simulink model "wlan_phy_tx_pmd"  (Simulink 7.8)
settings: Solver=VariableStepDiscrete  SolverMode=SingleTasking  StartTime=0.0  StopTime=inf  RelTol=1e-3
PostLoadFcn:
  | wlan_phy_tx_init
InitFcn:
  | wlan_phy_tx_init
StartFcn:
  | wlan_phy_tx_init
undefined symbols (not defined in the file): gcbh, ht_preamble_rom, MAX_CP_LEN, MAX_DATA_BITS_PER_SYM_PERIOD, MAX_NCBPS, MAX_NUM_BYTES, MAX_NUM_SC, MAX_NUM_SYMS, mcs_rom_11ag, mcs_rom_11n, Mod_Constellation_16QAM, Mod_Constellation_64QAM, Mod_Constellation_BPSK, Mod_Constellation_QPSK, Preamble_IQ, Preamble_IQ_scaled, tx_sim, wlan_tx_interleave_rom, xlBlockLoadCallback, xlGetNormalizedPeriod
libraries: xbsIndex_r4 x1358, xbsEDKLib_r4 x1
(part 8 of 10)

== system wlan_phy_tx_pmd/PSDU Syms Gen/Modulate/Control & Pilots/Data SC Map ==
  note: ROMs store mapping of subcarrier indexes as used by
      | upstream logic to subcarrier indexes into the IFFT. These
      | maps also encode which subcarriers are occupied.
      | Unoccupied subcarrier indexes are encoded as 64 in the
      | ROM (64 is an invalid subcarrier index).
      |
      | The mapping in these ROMs implements the effective
      | 'fftshift' from the 802.11 standard, where subcarriers are
      | loaded starting from the most negative subcarrier.
  Full Rate : Inport
  sc_ind : Inport  Port=2
  11a Subcarrier Map : xbsIndex_r4/ROM  depth=MAX_NUM_SC  initVector=sc_data_sym_map_11a  distributed_mem=Distributed memory  rst=off  init_reg=0  en=off  latency=0  gui_display_data_type=Fixed-point  arith_type=Unsigned  n_bits=ceil(log2(MAX_NUM_SC))+1  bin_pt=0  preci_type=Single  exp_width=8  frac_width=24  dbl_ovrd=off  optimize=Area  use_rpm=on  block_type=sprom
  11n HT20 Subcarrier Map : xbsIndex_r4/ROM  depth=MAX_NUM_SC  initVector=sc_data_sym_map_11n  distributed_mem=Distributed memory  rst=off  init_reg=0  en=off  latency=0  gui_display_data_type=Fixed-point  arith_type=Unsigned  n_bits=ceil(log2(MAX_NUM_SC))+1  bin_pt=0  preci_type=Single  exp_width=8  frac_width=24  dbl_ovrd=off  optimize=Area  use_rpm=on  block_type=sprom
  Constant2 : xbsIndex_r4/Constant  const=MAX_NUM_SC  gui_display_data_type=Fixed-point  arith_type=Unsigned  n_bits=ceil(log2(MAX_NUM_SC))+1  bin_pt=0  preci_type=Single  exp_width=8  frac_width=24  explicit_period=off  period=1  equ=P=C  opselect=C  inp2=PCIN>>17  opr=+  inp1=P  carry=CIN  dbl_ovrd=off  block_type=constant
  Logical : xbsIndex_r4/Logical  logical_function=AND  inputs=2  en=off  latency=0  precision=Full  arith_type=Unsigned  n_bits=16  bin_pt=0  align_bp=on  dbl_ovrd=off  block_type=logical
  Mux1 : xbsIndex_r4/Mux  inputs=2  en=off  latency=0  precision=Full  arith_type=Unsigned  n_bits=16  bin_pt=14  quantization=Truncate  overflow=Wrap  dbl_ovrd=off  block_type=mux
  Relational1 : xbsIndex_r4/Relational  mode=a!=b  en=off  latency=0  dbl_ovrd=off  block_type=relational
  Slice : xbsIndex_r4/Slice  nbits=ceil(log2(MAX_NUM_SC))  boolean_output=off  mode=Lower Bit Location + Width  bit1=0  base1=MSB of Input  bit0=0  base0=LSB of Input  dbl_ovrd=off  block_type=slice
  data_sym_ind : Outport
  data_sym_valid : Outport  Port=2
  wires:
  sc_ind/1 -> 11a Subcarrier Map/1, 11n HT20 Subcarrier Map/1
  Constant2/1 -> Relational1/2
  11a Subcarrier Map/1 -> Mux1/2
  11n HT20 Subcarrier Map/1 -> Mux1/3
  Logical/1 -> Mux1/1
  Mux1/1 -> Relational1/1, Slice/1
  Relational1/1 -> data_sym_valid/1
  [Tx_PHY_Mode_11n] -> Logical/1
  Full Rate/1 -> Logical/2
  Slice/1 -> data_sym_ind/1

== system wlan_phy_tx_pmd/PSDU Syms Gen/Modulate/Control & Pilots/Pilot Gen ==
  sc_ind : Inport
  reset : Inport  Port=2
  Pilot Shift : Inport  Port=3
  Constant1 : xbsIndex_r4/Constant  const=Mod_Constellation_BPSK(1)  gui_display_data_type=Fixed-point  arith_type=Signed (2's comp)  n_bits=12  bin_pt=11  preci_type=Single  exp_width=8  frac_width=24  explicit_period=off  period=1  equ=P=C  opselect=C  inp2=PCIN>>17  opr=+  inp1=P  carry=CIN  dbl_ovrd=off  block_type=constant
  Constant5 : xbsIndex_r4/Constant  const=Mod_Constellation_BPSK(2)  gui_display_data_type=Fixed-point  arith_type=Signed (2's comp)  n_bits=12  bin_pt=11  preci_type=Single  exp_width=8  frac_width=24  explicit_period=off  period=1  equ=P=C  opselect=C  inp2=PCIN>>17  opr=+  inp1=P  carry=CIN  dbl_ovrd=off  block_type=constant
  Delay : xbsIndex_r4/Delay  rst=off  infoeditControl=Selection of Reset will increase slice count due to use of real FFs and instead of SRLs  en=off  latency=1  dbl_ovrd=off  reg_retiming=off  block_type=delay
  Logical : xbsIndex_r4/Logical  logical_function=XOR  inputs=2  en=off  latency=0  precision=Full  arith_type=Unsigned  n_bits=8  bin_pt=2  align_bp=on  dbl_ovrd=off  block_type=logical
      settings: xl_area=[0, 0, 0, 0, 0, 0, 0]  block_version=VER_STRING_GOES_HERE
  Mux1 : xbsIndex_r4/Mux  inputs=2  en=off  latency=0  precision=Full  arith_type="Signed  (2's comp)"  n_bits=8  bin_pt=2  quantization=Truncate  overflow=Wrap  dbl_ovrd=off  block_type=mux
      settings: xl_area=[16 0 0 32 0 0 0]  block_version=VER_STRING_GOES_HERE
  Pilot Selection : Subsystem
  Posedge : Subsystem
  Relational1 : xbsIndex_r4/Relational  mode=a<b  en=off  latency=0  dbl_ovrd=off  block_type=relational
  Scrambling LFSR : Subsystem
  pilot_valid : Outport
  Pilot_I : Outport  Port=2
  wires:
  Pilot Selection/1(Pilot) -> pilot_valid/1
  Pilot Selection/2(Negate) -> Logical/1
  sc_ind/1 -> Pilot Selection/1(sc_ind), Delay/1, Relational1/1
  Delay/1 -> Relational1/2
  Relational1/1 -> Posedge/1(D)
  Posedge/1(Q) -> Scrambling LFSR/1(en)
  Scrambling LFSR/1(Q) -> Logical/2
  Logical/1 -> Mux1/1
  Constant5/1 -> Mux1/2
  Constant1/1 -> Mux1/3
  Mux1/1 -> Pilot_I/1
  reset/1 -> Scrambling LFSR/2(rst)
  Pilot Shift/1 -> Pilot Selection/2(Shift)

== system wlan_phy_tx_pmd/PSDU Syms Gen/Modulate/Control & Pilots/Posedge ==
  note: Rising Edge Detection
  D : Inport
  Delay : xbsIndex_r4/Delay  rst=off  infoeditControl=Selection of Reset will increase slice count due to use of real FFs and instead of SRLs  en=off  latency=1  dbl_ovrd=off  reg_retiming=off  block_type=delay
      settings: infoedit=Hardware notes: A delay line is a chain, each link of which is an SRL16 followed by a flip-flop. If register retiming is enabled, the delay line is a chain of flip-flops.  xl_area=[1 1 0 0 0 0 0]  block_version=VER_STRING_GOES_HERE
  Inverter : xbsIndex_r4/Inverter  en=off  latency=0  dbl_ovrd=off  block_type=inv
      settings: xl_area=[0 0 0 0 0 0 0]  block_version=VER_STRING_GOES_HERE
  Logical1 : xbsIndex_r4/Logical  logical_function=AND  inputs=2  en=off  latency=0  precision=Full  arith_type=Unsigned  n_bits=8  bin_pt=2  align_bp=on  dbl_ovrd=off  block_type=logical
      settings: xl_area=[1 0 0 1 0 0 0]  block_version=VER_STRING_GOES_HERE
  Q : Outport
  wires:
  D/1 -> Logical1/2, Delay/1
  Logical1/1 -> Q/1
  Inverter/1 -> Logical1/1
  Delay/1 -> Inverter/1

== system wlan_phy_tx_pmd/PSDU Syms Gen/Modulate/Control & Pilots/Posedge1 ==
  note: Rising Edge Detection
  D : Inport
  Delay : xbsIndex_r4/Delay  rst=off  infoeditControl=Selection of Reset will increase slice count due to use of real FFs and instead of SRLs  en=off  latency=1  dbl_ovrd=off  reg_retiming=off  block_type=delay
      settings: infoedit=Hardware notes: A delay line is a chain, each link of which is an SRL16 followed by a flip-flop. If register retiming is enabled, the delay line is a chain of flip-flops.  xl_area=[1 1 0 0 0 0 0]  block_version=VER_STRING_GOES_HERE
  Inverter : xbsIndex_r4/Inverter  en=off  latency=0  dbl_ovrd=off  block_type=inv
      settings: xl_area=[0 0 0 0 0 0 0]  block_version=VER_STRING_GOES_HERE
  Logical1 : xbsIndex_r4/Logical  logical_function=AND  inputs=2  en=off  latency=0  precision=Full  arith_type=Unsigned  n_bits=8  bin_pt=2  align_bp=on  dbl_ovrd=off  block_type=logical
      settings: xl_area=[1 0 0 1 0 0 0]  block_version=VER_STRING_GOES_HERE
  Q : Outport
  wires:
  Delay/1 -> Inverter/1
  Inverter/1 -> Logical1/1
  Logical1/1 -> Q/1
  D/1 -> Delay/1, Logical1/2

== system wlan_phy_tx_pmd/PSDU Syms Gen/Modulate/Control & Pilots/S-R Latch1 ==
  S : Inport
  R : Inport  Port=2
  Constant1 : xbsIndex_r4/Constant  const=1  gui_display_data_type=Fixed-point  arith_type=Boolean  n_bits=1  bin_pt=0  preci_type=Single  exp_width=8  frac_width=24  explicit_period=off  period=1  equ=P=C  opselect=C  inp2=PCIN>>17  opr=+  inp1=P  carry=CIN  dbl_ovrd=off  block_type=constant
      settings: block_version=VER_STRING_GOES_HERE
  Convert1 : xbsIndex_r4/Convert  gui_display_data_type=Boolean  arith_type=Boolean  n_bits=1  bin_pt=0  float_type=Single  exp_bits=8  fraction_bits=24  quantization=Truncate  overflow=Wrap  en=off  latency=0  dbl_ovrd=off  pipeline=off  block_type=convert
  Convert2 : xbsIndex_r4/Convert  gui_display_data_type=Boolean  arith_type=Boolean  n_bits=1  bin_pt=0  float_type=Single  exp_bits=8  fraction_bits=24  quantization=Truncate  overflow=Wrap  en=off  latency=0  dbl_ovrd=off  pipeline=off  block_type=convert
  Register2 : xbsIndex_r4/Register  init=0  rst=on  en=on  dbl_ovrd=off  block_type=register
      settings: xl_area=[1 1 0 0 0 0 0]  block_version=VER_STRING_GOES_HERE
  Q : Outport
  wires:
  Convert2/1 -> Register2/3
  Convert1/1 -> Register2/2
  Constant1/1 -> Register2/1
  R/1 -> Convert1/1
  Register2/1 -> Q/1
  S/1 -> Convert2/1

== system wlan_phy_tx_pmd/PSDU Syms Gen/Modulate/Control & Pilots/Subcarrier Index Count ==
  en : Inport
  reset : Inport  Port=2
  AddSub : xbsIndex_r4/AddSub  mode=Subtraction  use_carryin=off  use_carryout=off  en=off  latency=0  precision=Full  arith_type=Unsigned  n_bits=16  bin_pt=14  quantization=Truncate  overflow=Wrap  dbl_ovrd=off  use_behavioral_HDL=off  hw_selection=Fabric  pipelined=off  block_type=addsub
  Constant1 : xbsIndex_r4/Constant  const=1  gui_display_data_type=Fixed-point  arith_type=Unsigned  n_bits=1  bin_pt=0  preci_type=Single  exp_width=8  frac_width=24  explicit_period=off  period=1  equ=P=C  opselect=C  inp2=PCIN>>17  opr=+  inp1=P  carry=CIN  dbl_ovrd=off  block_type=constant
  Logical1 : xbsIndex_r4/Logical  logical_function=AND  inputs=2  en=off  latency=0  precision=Full  arith_type=Unsigned  n_bits=16  bin_pt=0  align_bp=on  dbl_ovrd=off  block_type=logical
  Logical2 : xbsIndex_r4/Logical  logical_function=OR  inputs=2  en=off  latency=0  precision=Full  arith_type=Unsigned  n_bits=16  bin_pt=0  align_bp=on  dbl_ovrd=off  block_type=logical
  Relational3 : xbsIndex_r4/Relational  mode=a=b  en=off  latency=0  dbl_ovrd=off  block_type=relational
  Subcarrier Index : xbsIndex_r4/Counter  cnt_type=Free Running  cnt_to=47  operation=Up  start_count=0  cnt_by_val=1  arith_type=Unsigned  n_bits=ceil(log2(MAX_NUM_SC))  bin_pt=0  load_pin=off  rst=on  en=on  explicit_period=off  period=4  dbl_ovrd=off  use_behavioral_HDL=off  implementation=Fabric  block_type=counter
  sc_ind : Outport
  last : Outport  Port=2
  wires:
  Subcarrier Index/1 -> Relational3/2, sc_ind/1
  AddSub/1 -> Relational3/1
  Relational3/1 -> Logical1/1
  en/1 -> Subcarrier Index/2, Logical1/2
  Logical2/1 -> Subcarrier Index/1
  reset/1 -> Logical2/1
  Logical1/1 -> Logical2/2, last/1
  [regTx_NUM_SC] -> AddSub/1
  Constant1/1 -> AddSub/2

== system wlan_phy_tx_pmd/PSDU Syms Gen/Pkt Data/BRAM IF 64b/BRAM Addr Map ==
  note: OFDM Byte Index Tx -> Memory mapping
      | 11a/g Tx
      |
      | T=Tx byte index
      | M=Memory byte index
      |
      | T  M
      | 0  0   SIGNAL[0]
      | 1  1   SIGNAL[1]
      | 2  2   SIGNAL[2]
      | 3  3   SERVICE[0]
      | 4  4   SERVICE[1]
      |    5   no read
      |    ...
      |    15   no read
      | 5  16  MPDU[0]
      | 6  17  MPDU[1]
      | ...
  note: OFDM Byte Index Tx -> Memory mapping
      | 11n/ac Tx
      |
      | T=Rx byte index
      | M=Memory byte index
      |
      | T  M
      | 0  0   SIGNAL[0]
      | 1  1   SIGNAL[1]
      | 2  2   SIGNAL[2]
      | 3  3   HT-SIG[0]
      | 4  4   HT-SIG[1]
      | 5  5   HT-SIG[2]
      | 6  6   HT-SIG[3]
      | 7  7   HT-SIG[4]
      | 8  8   HT-SIG[5]
      | 9  9   SERVICE[0]
      | 10 10  SERVICE[1]
      |    11  no read
      | ...
      |    15  no read
      | 11 16  MAC Payload[0]
      | 12 17  MAC Payload[1]
      | ...
  note: Packet buffer contents depend on the PHY mode. 11n payloads
      | must include the HTSIG field, for example. For easier addressing
      | in software the Tx PHY logic uses the address mapping below. Note
      | that the MAC payload always starts at a 64-bit aligned address. This
      | allows efficient use of the DMA in CPU high to move MAC payloads into
      | the packet buffer. CPU Low adds the PHY-mode-specific fields before
      | transmission.
      |
      | The MAC code must write valid bytes for SIGNAL, HT-SIG and SERVICE
      | fields. The PHY will abort if the SIGNAL or HT-SIG fields are invlid.
      | The MAC software must set the SERVICE field bytes to 0 to ensure
      | the resulting payload can be de-scrambled by the receiver.
  Tx Ind : Inport
  AddSub1 : xbsIndex_r4/AddSub  mode=Addition  use_carryin=off  use_carryout=off  en=off  latency=0  precision=User Defined  arith_type=Unsigned  n_bits=ceil(log2(MAX_NUM_BYTES))  bin_pt=0  quantization=Truncate  overflow=Wrap  dbl_ovrd=off  use_behavioral_HDL=off  hw_selection=Fabric  pipelined=off  block_type=addsub
  Constant1 : xbsIndex_r4/Constant  const=4  gui_display_data_type=Fixed-point  arith_type=Unsigned  n_bits=3  bin_pt=0  preci_type=Single  exp_width=8  frac_width=24  explicit_period=off  period=1  equ=P=C  opselect=C  inp2=PCIN>>17  opr=+  inp1=P  carry=CIN  dbl_ovrd=off  block_type=constant
  Constant2 : xbsIndex_r4/Constant  const=11  gui_display_data_type=Fixed-point  arith_type=Unsigned  n_bits=4  bin_pt=0  preci_type=Single  exp_width=8  frac_width=24  explicit_period=off  period=1  equ=P=C  opselect=C  inp2=PCIN>>17  opr=+  inp1=P  carry=CIN  dbl_ovrd=off  block_type=constant
  Constant3 : xbsIndex_r4/Constant  const=10  gui_display_data_type=Fixed-point  arith_type=Unsigned  n_bits=4  bin_pt=0  preci_type=Single  exp_width=8  frac_width=24  explicit_period=off  period=1  equ=P=C  opselect=C  inp2=PCIN>>17  opr=+  inp1=P  carry=CIN  dbl_ovrd=off  block_type=constant
  Constant4 : xbsIndex_r4/Constant  const=5  gui_display_data_type=Fixed-point  arith_type=Unsigned  n_bits=3  bin_pt=0  preci_type=Single  exp_width=8  frac_width=24  explicit_period=off  period=1  equ=P=C  opselect=C  inp2=PCIN>>17  opr=+  inp1=P  carry=CIN  dbl_ovrd=off  block_type=constant
  Mux1 : xbsIndex_r4/Mux  inputs=2  en=off  latency=0  precision=Full  arith_type=Unsigned  n_bits=16  bin_pt=14  quantization=Truncate  overflow=Wrap  dbl_ovrd=off  block_type=mux
  Mux2 : xbsIndex_r4/Mux  inputs=2  en=off  latency=0  precision=Full  arith_type=Unsigned  n_bits=16  bin_pt=14  quantization=Truncate  overflow=Wrap  dbl_ovrd=off  block_type=mux
  Mux5 : xbsIndex_r4/Mux  inputs=2  en=off  latency=0  precision=Full  arith_type=Unsigned  n_bits=16  bin_pt=14  quantization=Truncate  overflow=Wrap  dbl_ovrd=off  block_type=mux
  Relational : xbsIndex_r4/Relational  mode=a<=b  en=off  latency=0  dbl_ovrd=off  block_type=relational
  Mem Addr : Outport
  wires:
  Mux2/1 -> AddSub1/2
  Tx Ind/1 -> Relational/1, AddSub1/1, Mux5/3
  Relational/1 -> Mux5/1
  Mux5/1 -> Mem Addr/1
  AddSub1/1 -> Mux5/2
  [Tx_PHY_Mode_11n_ac] -> Mux1/1, Mux2/1
  Constant1/1 -> Mux1/2
  Mux1/1 -> Relational/2
  Constant2/1 -> Mux2/2
  Constant3/1 -> Mux1/3
  Constant4/1 -> Mux2/3

== system wlan_phy_tx_pmd/PSDU Syms Gen/Pkt Data/BRAM IF 64b/BRAM Interface ==
  Pkt Buf Index : Inport
  64b Word Addr : Inport  Port=2
  BRAM_Addr : xbsIndex_r4/Gateway Out  inherit_from_input=off  hdl_port=on  timing_constraint=None  locs_specified=off  LOCs={}  UseAsDAC=off  DACChannel='1'  block_type=gatewayout
      settings: infoedit="Gateway out block.  Converts Xilinx fixed point inputs into ouputs of type Simulink integer, double, or fixed point.<P><P>Hardware notes:  In hardware these blocks become top level output ports or are discarded, depending on how they are configured."  xl_area=[0, 0, 0, 0, 0, 0, 0]  block_version=VER_STRING_GOES_HERE
  BRAM_Din : xbsIndex_r4/Gateway In  gui_display_data_type=Fixed-point  arith_type=Unsigned  n_bits=64  bin_pt=0  preci_type=Single  exp_width=8  frac_width=24  quantization="Round  (unbiased: +/- Inf)"  overflow=Saturate  period=1  dbl_ovrd=off  timing_constraint=None  locs_specified=off  LOCs={}  UseAsADC=off  ADCChannel='1'  inherit_from_input=off  hdl_port=on  block_type=gatewayin
      settings: block_version=VER_STRING_GOES_HERE
  BRAM_Dout : xbsIndex_r4/Gateway Out  inherit_from_input=off  hdl_port=on  timing_constraint=None  locs_specified=off  LOCs={}  UseAsDAC=off  DACChannel='1'  block_type=gatewayout
      settings: infoedit="Gateway out block.  Converts Xilinx fixed point inputs into ouputs of type Simulink integer, double, or fixed point.<P><P>Hardware notes:  In hardware these blocks become top level output ports or are discarded, depending on how they are configured."  xl_area=[0, 0, 0, 0, 0, 0, 0]  block_version=VER_STRING_GOES_HERE
  BRAM_En : xbsIndex_r4/Gateway Out  inherit_from_input=off  hdl_port=on  timing_constraint=None  locs_specified=off  LOCs={}  UseAsDAC=off  DACChannel='1'  block_type=gatewayout
      settings: infoedit="Gateway out block.  Converts Xilinx fixed point inputs into ouputs of type Simulink integer, double, or fixed point.<P><P>Hardware notes:  In hardware these blocks become top level output ports or are discarded, depending on how they are configured."  block_version=8.2.02
  BRAM_Reset : xbsIndex_r4/Gateway Out  inherit_from_input=off  hdl_port=on  timing_constraint=None  locs_specified=off  LOCs={}  UseAsDAC=off  DACChannel='1'  block_type=gatewayout
      settings: infoedit="Gateway out block.  Converts Xilinx fixed point inputs into ouputs of type Simulink integer, double, or fixed point.<P><P>Hardware notes:  In hardware these blocks become top level output ports or are discarded, depending on how they are configured."  block_version=8.2.02
  BRAM_WEn : xbsIndex_r4/Gateway Out  inherit_from_input=off  hdl_port=on  timing_constraint=None  locs_specified=off  LOCs={}  UseAsDAC=off  DACChannel='1'  block_type=gatewayout
      settings: infoedit="Gateway out block.  Converts Xilinx fixed point inputs into ouputs of type Simulink integer, double, or fixed point.<P><P>Hardware notes:  In hardware these blocks become top level output ports or are discarded, depending on how they are configured."  xl_area=[0, 0, 0, 0, 0, 0, 0]  block_version=VER_STRING_GOES_HERE
  Concat : xbsIndex_r4/Concat  num_inputs=4  dbl_ovrd=off  block_type=concat
  Constant : Constant  Value=0
  Constant1 : xbsIndex_r4/Constant  const=1  gui_display_data_type=Fixed-point  arith_type=Unsigned  n_bits=1  bin_pt=0  preci_type=Single  exp_width=8  frac_width=24  explicit_period=on  period=1  equ=P=C  opselect=C  inp2=PCIN>>17  opr=+  inp1=P  carry=CIN  dbl_ovrd=off  block_type=constant
      settings: block_version=8.2.02
  Constant2 : xbsIndex_r4/Constant  const=0  gui_display_data_type=Fixed-point  arith_type=Unsigned  n_bits=1  bin_pt=0  preci_type=Single  exp_width=8  frac_width=24  explicit_period=on  period=1  equ=P=C  opselect=C  inp2=PCIN>>17  opr=+  inp1=P  carry=CIN  dbl_ovrd=off  block_type=constant
      settings: block_version=8.2.02
  Constant3 : xbsIndex_r4/Constant  const=0  gui_display_data_type=Fixed-point  arith_type=Unsigned  n_bits=3  bin_pt=0  preci_type=Single  exp_width=8  frac_width=24  explicit_period=off  period=1  equ=P=C  opselect=C  inp2=PCIN>>17  opr=+  inp1=P  carry=CIN  dbl_ovrd=off  block_type=constant
  Constant4 : xbsIndex_r4/Constant  const=0  gui_display_data_type=Fixed-point  arith_type=Unsigned  n_bits=16  bin_pt=0  preci_type=Single  exp_width=8  frac_width=24  explicit_period=off  period=1  equ=P=C  opselect=C  inp2=PCIN>>17  opr=+  inp1=P  carry=CIN  dbl_ovrd=off  block_type=constant
  Constant7 : xbsIndex_r4/Constant  const=0  gui_display_data_type=Fixed-point  arith_type=Unsigned  n_bits=64  bin_pt=0  preci_type=Single  exp_width=8  frac_width=24  explicit_period=on  period=1  equ=P=C  opselect=C  inp2=PCIN>>17  opr=+  inp1=P  carry=CIN  dbl_ovrd=off  block_type=constant
      settings: block_version=8.2.02
  Constant8 : xbsIndex_r4/Constant  const=0  gui_display_data_type=Fixed-point  arith_type=Unsigned  n_bits=8  bin_pt=0  preci_type=Single  exp_width=8  frac_width=24  explicit_period=on  period=1  equ=P=C  opselect=C  inp2=PCIN>>17  opr=+  inp1=P  carry=CIN  dbl_ovrd=off  block_type=constant
      settings: block_version=8.2.02
  Sim RAM : Subsystem
  Simulation Multiplexer : xbsIndex_r4/Simulation Multiplexer  sim_sel=1  hw_sel=2  block_type=simmux
      settings: infoedit="Distinguish input subsystems as \"simulation only\" and \"generation only\".  The input specified For Simulation will be used during Simulink simulation.  The input specified For Generation will be used during code generation.  This block will typically be used on the output of a HW Co-Simulation, Black Box, or ModelSim subsystem.<br><br>Hardware Notes: This block costs nothing."
  Terminator{,2..5} (5 alike) : Terminator
  64b Data : Outport
  wires:
  Sim RAM/1(64b) -> Simulation Multiplexer/1
  BRAM_Din/1 -> Simulation Multiplexer/2
  BRAM_WEn/1 -> Terminator5/1
  BRAM_Reset/1 -> Terminator4/1
  BRAM_En/1 -> Terminator3/1
  BRAM_Dout/1 -> Terminator2/1
  BRAM_Addr/1 -> Terminator/1
  Constant2/1 -> BRAM_Reset/1
  Constant1/1 -> BRAM_En/1
  Constant/1 -> BRAM_Din/1
  Constant7/1 -> BRAM_Dout/1
  Constant8/1 -> BRAM_WEn/1
  64b Word Addr/1 -> Sim RAM/1(Addr), Concat/3
  Constant3/1 -> Concat/4
  Constant4/1 -> Concat/1
  Concat/1 -> BRAM_Addr/1
  Simulation Multiplexer/1 -> 64b Data/1
  Pkt Buf Index/1 -> Concat/2

== system wlan_phy_tx_pmd/PSDU Syms Gen/Pkt Data/BRAM IF 64b/Byte Sel ==
  64b : Inport
  B Sel : Inport  Port=2
  B0 : xbsIndex_r4/Slice  nbits=8  boolean_output=off  mode=Lower Bit Location + Width  bit1=0  base1=MSB of Input  bit0=0  base0=LSB of Input  dbl_ovrd=off  block_type=slice
  B1 : xbsIndex_r4/Slice  nbits=8  boolean_output=off  mode=Lower Bit Location + Width  bit1=0  base1=MSB of Input  bit0=8  base0=LSB of Input  dbl_ovrd=off  block_type=slice
  B2 : xbsIndex_r4/Slice  nbits=8  boolean_output=off  mode=Lower Bit Location + Width  bit1=0  base1=MSB of Input  bit0=16  base0=LSB of Input  dbl_ovrd=off  block_type=slice
  B3 : xbsIndex_r4/Slice  nbits=8  boolean_output=off  mode=Lower Bit Location + Width  bit1=0  base1=MSB of Input  bit0=24  base0=LSB of Input  dbl_ovrd=off  block_type=slice
  B4 : xbsIndex_r4/Slice  nbits=8  boolean_output=off  mode=Lower Bit Location + Width  bit1=0  base1=MSB of Input  bit0=32  base0=LSB of Input  dbl_ovrd=off  block_type=slice
  B5 : xbsIndex_r4/Slice  nbits=8  boolean_output=off  mode=Lower Bit Location + Width  bit1=0  base1=MSB of Input  bit0=40  base0=LSB of Input  dbl_ovrd=off  block_type=slice
  B6 : xbsIndex_r4/Slice  nbits=8  boolean_output=off  mode=Lower Bit Location + Width  bit1=0  base1=MSB of Input  bit0=48  base0=LSB of Input  dbl_ovrd=off  block_type=slice
  B7 : xbsIndex_r4/Slice  nbits=8  boolean_output=off  mode=Lower Bit Location + Width  bit1=0  base1=MSB of Input  bit0=56  base0=LSB of Input  dbl_ovrd=off  block_type=slice
  Mux : xbsIndex_r4/Mux  inputs=8  en=off  latency=0  precision=Full  arith_type=Unsigned  n_bits=16  bin_pt=14  quantization=Truncate  overflow=Wrap  dbl_ovrd=off  block_type=mux
  B : Outport
  wires:
  Mux/1 -> B/1
  B Sel/1 -> Mux/1
  64b/1 -> B2/1, B3/1, B4/1, B5/1, B6/1, B7/1, B1/1, B0/1
  B3/1 -> Mux/5
  B2/1 -> Mux/4
  B1/1 -> Mux/3
  B0/1 -> Mux/2
  B4/1 -> Mux/6
  B5/1 -> Mux/7
  B6/1 -> Mux/8
  B7/1 -> Mux/9

== system wlan_phy_tx_pmd/PSDU Syms Gen/Pkt Data/FCS Calc/Byte Sel ==
  32b : Inport
  B Sel : Inport  Port=2
  B0 : xbsIndex_r4/Slice  nbits=8  boolean_output=off  mode=Lower Bit Location + Width  bit1=0  base1=MSB of Input  bit0=0  base0=LSB of Input  dbl_ovrd=off  block_type=slice
  B1 : xbsIndex_r4/Slice  nbits=8  boolean_output=off  mode=Lower Bit Location + Width  bit1=0  base1=MSB of Input  bit0=8  base0=LSB of Input  dbl_ovrd=off  block_type=slice
  B2 : xbsIndex_r4/Slice  nbits=8  boolean_output=off  mode=Lower Bit Location + Width  bit1=0  base1=MSB of Input  bit0=16  base0=LSB of Input  dbl_ovrd=off  block_type=slice
  B3 : xbsIndex_r4/Slice  nbits=8  boolean_output=off  mode=Lower Bit Location + Width  bit1=0  base1=MSB of Input  bit0=24  base0=LSB of Input  dbl_ovrd=off  block_type=slice
  Constant : xbsIndex_r4/Constant  const=hex2dec('87654321') %hex2dec('FF00FF00') %  gui_display_data_type=Fixed-point  arith_type=Unsigned  n_bits=32  bin_pt=0  preci_type=Single  exp_width=8  frac_width=24  explicit_period=on  period=1  equ=P=C  opselect=C  inp2=PCIN>>17  opr=+  inp1=P  carry=CIN  dbl_ovrd=off  block_type=constant
  Mux : xbsIndex_r4/Mux  inputs=4  en=off  latency=0  precision=Full  arith_type=Unsigned  n_bits=16  bin_pt=14  quantization=Truncate  overflow=Wrap  dbl_ovrd=off  block_type=mux
  B : Outport
  wires:
  Mux/1 -> B/1
  B Sel/1 -> Mux/1
  32b/1 -> B0/1, B1/1, B2/1, B3/1
  B0/1 -> Mux/5
  B1/1 -> Mux/4
  B2/1 -> Mux/3
  B3/1 -> Mux/2

== system wlan_phy_tx_pmd/PSDU Syms Gen/Pkt Data/FCS Calc/CRC32 Calc ==
  byte : Inport
  en : Inport  Port=2
  24LSB : xbsIndex_r4/Slice  nbits=24  boolean_output=off  mode=Lower Bit Location + Width  bit1=0  base1=MSB of Input  bit0=0  base0=LSB of Input  dbl_ovrd=off  block_type=slice
      settings: infoedit="Extracts a given range of bits from each input sample and presents it at the output.  The output type is ordinarily unsigned with binary point at zero, but can be Boolean when the slice is one bit wide.<P><P>Hardware notes: In hardware this block costs nothing."  block_version=VER_STRING_GOES_HERE
  8MSB : xbsIndex_r4/Slice  nbits=8  boolean_output=off  mode=Upper Bit Location + Width  bit1=0  base1=MSB of Input  bit0=0  base0=LSB of Input  dbl_ovrd=off  block_type=slice
      settings: infoedit="Extracts a given range of bits from each input sample and presents it at the output.  The output type is ordinarily unsigned with binary point at zero, but can be Boolean when the slice is one bit wide.<P><P>Hardware notes: In hardware this block costs nothing."  block_version=VER_STRING_GOES_HERE
  Assert : xbsIndex_r4/Assert  assert_type=off  type_source=Explicitly  gui_display_data_type=Fixed-point  arith_type="Signed  (2's comp)"  n_bits=16  bin_pt=14  preci_type=Single  exp_width=8  frac_width=24  assert_rate=on  rate_source=Explicitly  period=1  output_port=on  block_type=assert
  Assert1 : xbsIndex_r4/Assert  assert_type=off  type_source=Explicitly  gui_display_data_type=Fixed-point  arith_type="Signed  (2's comp)"  n_bits=16  bin_pt=14  preci_type=Single  exp_width=8  frac_width=24  assert_rate=on  rate_source=Explicitly  period=1  output_port=on  block_type=assert
      settings: block_version=VER_STRING_GOES_HERE
  B0 : xbsIndex_r4/Slice  nbits=8  boolean_output=off  mode=Lower Bit Location + Width  bit1=0  base1=MSB of Input  bit0=0  base0=LSB of Input  dbl_ovrd=off  block_type=slice
  B1 : xbsIndex_r4/Slice  nbits=8  boolean_output=off  mode=Lower Bit Location + Width  bit1=0  base1=MSB of Input  bit0=8  base0=LSB of Input  dbl_ovrd=off  block_type=slice
  B2 : xbsIndex_r4/Slice  nbits=8  boolean_output=off  mode=Lower Bit Location + Width  bit1=0  base1=MSB of Input  bit0=16  base0=LSB of Input  dbl_ovrd=off  block_type=slice
  B3 : xbsIndex_r4/Slice  nbits=8  boolean_output=off  mode=Lower Bit Location + Width  bit1=0  base1=MSB of Input  bit0=24  base0=LSB of Input  dbl_ovrd=off  block_type=slice
  CRC Remainders1 : xbsIndex_r4/ROM  depth=256  initVector=CRC_Table32  distributed_mem=Distributed memory  rst=off  init_reg=0  en=off  latency=0  gui_display_data_type=Fixed-point  arith_type=Unsigned  n_bits=32  bin_pt=0  preci_type=Single  exp_width=8  frac_width=24  dbl_ovrd=off  optimize=Area  use_rpm=off  block_type=sprom
      settings: xl_area=[0, 0, 0, 0, 0, 0, 0]  block_version=VER_STRING_GOES_HERE
  Concat : xbsIndex_r4/Concat  num_inputs=4  dbl_ovrd=off  block_type=concat
  Concat1 : xbsIndex_r4/Concat  num_inputs=2  dbl_ovrd=off  block_type=concat
      settings: block_version=VER_STRING_GOES_HERE
  Constant1 : xbsIndex_r4/Constant  const=0  gui_display_data_type=Fixed-point  arith_type=Unsigned  n_bits=8  bin_pt=0  preci_type=Single  exp_width=8  frac_width=24  explicit_period=off  period=1  equ=P=C  opselect=C  inp2=PCIN>>17  opr=+  inp1=P  carry=CIN  dbl_ovrd=off  block_type=constant
      settings: block_version=VER_STRING_GOES_HERE
  Endian Swap : Subsystem
  Endian Swap1 : Subsystem
  Endian Swap2 : Subsystem
  Endian Swap3 : Subsystem
  Endian Swap4 : Subsystem
  Inverter : xbsIndex_r4/Inverter  en=off  latency=0  dbl_ovrd=off  block_type=inv
  Logical3 : xbsIndex_r4/Logical  logical_function=XOR  inputs=2  en=off  latency=0  precision=Full  arith_type=Unsigned  n_bits=8  bin_pt=2  align_bp=on  dbl_ovrd=off  block_type=logical
      settings: xl_area=[0, 0, 0, 0, 0, 0, 0]  block_version=VER_STRING_GOES_HERE
  Logical4 : xbsIndex_r4/Logical  logical_function=XOR  inputs=2  en=off  latency=0  precision=Full  arith_type=Unsigned  n_bits=8  bin_pt=2  align_bp=on  dbl_ovrd=off  block_type=logical
      settings: xl_area=[0, 0, 0, 0, 0, 0, 0]  block_version=VER_STRING_GOES_HERE
  crc_accum : xbsIndex_r4/Register  init=hex2dec('FFFFFFFF')  rst=on  en=on  dbl_ovrd=off  block_type=register
      settings: xl_area=[0, 0, 0, 0, 0, 0, 0]  block_version=VER_STRING_GOES_HERE
  CRC32 : Outport
  wires:
  Inverter/1 -> B0/1, B1/1, B3/1, B2/1
  Endian Swap4/1(I) -> Concat/4
  Endian Swap3/1(I) -> Concat/3
  Endian Swap2/1(I) -> Concat/2
  Endian Swap1/1(I) -> Concat/1
  Endian Swap/1(I) -> Logical3/2
  Concat/1 -> Assert/1
  B3/1 -> Endian Swap4/1(B)
  B2/1 -> Endian Swap3/1(B)
  B1/1 -> Endian Swap2/1(B)
  B0/1 -> Endian Swap1/1(B)
  byte/1 -> Endian Swap/1(B)
  8MSB/1 -> Logical3/1
  24LSB/1 -> Concat1/1
  [TX_RESET] -> crc_accum/2
  Assert1/1 -> Inverter/1, 8MSB/1, 24LSB/1
  crc_accum/1 -> Assert1/1
  Logical4/1 -> crc_accum/1
  Constant1/1 -> Concat1/2
  Concat1/1 -> Logical4/1
  CRC Remainders1/1 -> Logical4/2
  Logical3/1 -> CRC Remainders1/1
  Assert/1 -> CRC32/1
  en/1 -> crc_accum/3

== system wlan_phy_tx_pmd/PSDU Syms Gen/Pkt Data/FCS Calc/posedge ==
  D : Inport
  Delay : xbsIndex_r4/Delay  rst=off  infoeditControl=Selection of Reset will increase slice count due to use of real FFs and instead of SRLs  en=off  latency=1  dbl_ovrd=off  reg_retiming=off  block_type=delay
      settings: infoedit=Hardware notes: A delay line is a chain, each link of which is an SRL16 followed by a flip-flop. If register retiming is enabled, the delay line is a chain of flip-flops.  xl_area=[1 1 0 0 0 0 0]  block_version=VER_STRING_GOES_HERE
  Inverter : xbsIndex_r4/Inverter  en=off  latency=0  dbl_ovrd=off  block_type=inv
      settings: xl_area=[0 0 0 0 0 0 0]  block_version=VER_STRING_GOES_HERE
  Logical1 : xbsIndex_r4/Logical  logical_function=AND  inputs=2  en=off  latency=0  precision=Full  arith_type=Unsigned  n_bits=8  bin_pt=2  align_bp=on  dbl_ovrd=off  block_type=logical
      settings: xl_area=[1 0 0 1 0 0 0]  block_version=VER_STRING_GOES_HERE
  Q : Outport
  wires:
  Logical1/1 -> Q/1
  D/1 -> Delay/1, Logical1/1
  Delay/1 -> Inverter/1
  Inverter/1 -> Logical1/2

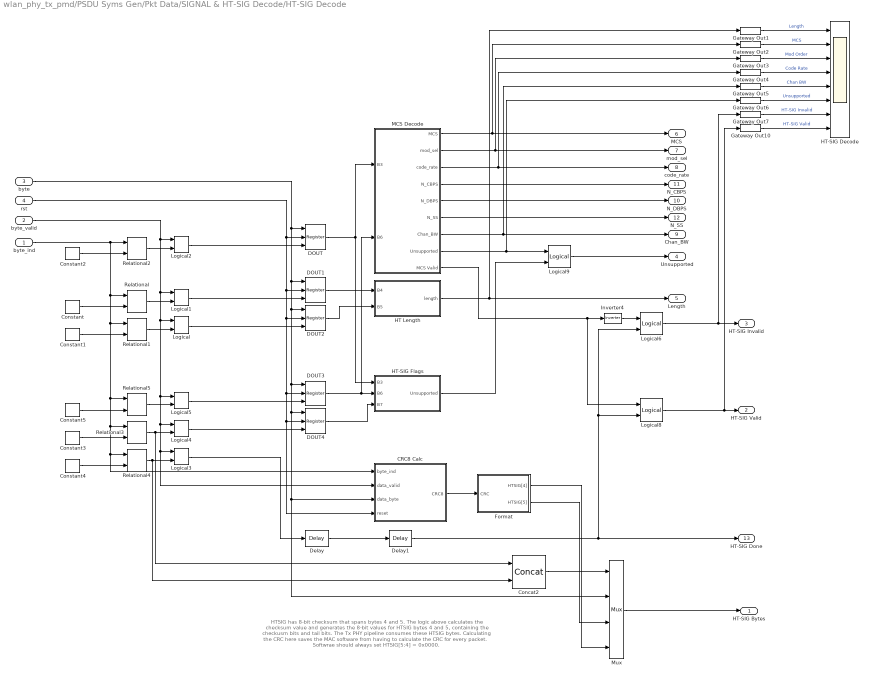
== system wlan_phy_tx_pmd/PSDU Syms Gen/Pkt Data/SIGNAL & HT-SIG Decode/HT-SIG Decode ==
  note: HTSIG has 8-bit checksum that spans bytes 4 and 5. The logic above
      | calculates the checksum value and generates the 8-bit values for HTSIG
      | bytes 4 and 5, containing the checkusm bits and tail bits. The Tx PHY
      | pipeline consumes these HTSIG bytes. Calculating the CRC here saves
      | the MAC software from having to calculate the CRC for every packet.
      |
      | Softwrae should always set HTSIG[5:4] = 0x0000.
  byte_ind : Inport
  byte_valid : Inport  Port=2
  byte : Inport  Port=3
  rst : Inport  Port=4
  CRC8 Calc : Subsystem
  Concat2 : xbsIndex_r4/Concat  num_inputs=2  dbl_ovrd=off  block_type=concat
  Constant : xbsIndex_r4/Constant  const=4  gui_display_data_type=Fixed-point  arith_type=Unsigned  n_bits=3  bin_pt=0  preci_type=Single  exp_width=8  frac_width=24  explicit_period=off  period=1  equ=P=C  opselect=C  inp2=PCIN>>17  opr=+  inp1=P  carry=CIN  dbl_ovrd=off  block_type=constant
  Constant1 : xbsIndex_r4/Constant  const=5  gui_display_data_type=Fixed-point  arith_type=Unsigned  n_bits=3  bin_pt=0  preci_type=Single  exp_width=8  frac_width=24  explicit_period=off  period=1  equ=P=C  opselect=C  inp2=PCIN>>17  opr=+  inp1=P  carry=CIN  dbl_ovrd=off  block_type=constant
  Constant2 : xbsIndex_r4/Constant  const=3  gui_display_data_type=Fixed-point  arith_type=Unsigned  n_bits=2  bin_pt=0  preci_type=Single  exp_width=8  frac_width=24  explicit_period=off  period=1  equ=P=C  opselect=C  inp2=PCIN>>17  opr=+  inp1=P  carry=CIN  dbl_ovrd=off  block_type=constant
  Constant3 : xbsIndex_r4/Constant  const=7  gui_display_data_type=Fixed-point  arith_type=Unsigned  n_bits=3  bin_pt=0  preci_type=Single  exp_width=8  frac_width=24  explicit_period=off  period=1  equ=P=C  opselect=C  inp2=PCIN>>17  opr=+  inp1=P  carry=CIN  dbl_ovrd=off  block_type=constant
  Constant4 : xbsIndex_r4/Constant  const=8  gui_display_data_type=Fixed-point  arith_type=Unsigned  n_bits=4  bin_pt=0  preci_type=Single  exp_width=8  frac_width=24  explicit_period=off  period=1  equ=P=C  opselect=C  inp2=PCIN>>17  opr=+  inp1=P  carry=CIN  dbl_ovrd=off  block_type=constant
  Constant5 : xbsIndex_r4/Constant  const=6  gui_display_data_type=Fixed-point  arith_type=Unsigned  n_bits=3  bin_pt=0  preci_type=Single  exp_width=8  frac_width=24  explicit_period=off  period=1  equ=P=C  opselect=C  inp2=PCIN>>17  opr=+  inp1=P  carry=CIN  dbl_ovrd=off  block_type=constant
  DOUT : xbsIndex_r4/Register  init=0  rst=on  en=on  dbl_ovrd=off  block_type=register
  DOUT1 : xbsIndex_r4/Register  init=100  rst=on  en=on  dbl_ovrd=off  block_type=register
  DOUT2 : xbsIndex_r4/Register  init=0  rst=on  en=on  dbl_ovrd=off  block_type=register
  DOUT3 : xbsIndex_r4/Register  init=hex2dec('03')  rst=on  en=on  dbl_ovrd=off  block_type=register
  DOUT4 : xbsIndex_r4/Register  init=hex2dec('E0')  rst=on  en=on  dbl_ovrd=off  block_type=register
  Delay : xbsIndex_r4/Delay  rst=off  infoeditControl=Selection of Reset will increase slice count due to use of real FFs and instead of SRLs  en=off  latency=1  dbl_ovrd=off  reg_retiming=off  block_type=delay
  Delay1 : xbsIndex_r4/Delay  rst=off  infoeditControl=Selection of Reset will increase slice count due to use of real FFs and instead of SRLs  en=off  latency=1  dbl_ovrd=off  reg_retiming=off  block_type=delay
  Format : Subsystem
  Gateway Out{1..7,10} (8 alike) : xbsIndex_r4/Gateway Out  inherit_from_input=off  hdl_port=off  timing_constraint=None  locs_specified=off  LOCs={}  UseAsDAC=off  DACChannel='1'  block_type=gatewayout
  HT Length : Subsystem
  HT-SIG Decode : Scope  NumInputPorts=8
      settings: TimeRange=7000  YMin=0~0~0~0~100~-1~-1~-1  YMax=1~1~150~1~300~1~1~1  SaveName=ScopeData45
  HT-SIG Flags : Subsystem
  Inverter4 : xbsIndex_r4/Inverter  en=off  latency=0  dbl_ovrd=off  block_type=inv
  Logical{,1..6,8} (8 alike) : xbsIndex_r4/Logical  logical_function=AND  inputs=2  en=off  latency=0  precision=Full  arith_type=Unsigned  n_bits=16  bin_pt=0  align_bp=on  dbl_ovrd=off  block_type=logical
  Logical9 : xbsIndex_r4/Logical  logical_function=OR  inputs=2  en=off  latency=0  precision=Full  arith_type=Unsigned  n_bits=16  bin_pt=0  align_bp=on  dbl_ovrd=off  block_type=logical
  MCS Decode : Subsystem
  Mux : xbsIndex_r4/Mux  inputs=3  en=off  latency=0  precision=Full  arith_type=Unsigned  n_bits=16  bin_pt=14  quantization=Truncate  overflow=Wrap  dbl_ovrd=off  block_type=mux
  Relational{,1..5} (6 alike) : xbsIndex_r4/Relational  mode=a=b  en=off  latency=0  dbl_ovrd=off  block_type=relational
  HT-SIG Bytes : Outport
  HT-SIG Valid : Outport  Port=2
  HT-SIG Invalid : Outport  Port=3
  Unsupported : Outport  Port=4
  Length : Outport  Port=5
  MCS : Outport  Port=6
  mod_sel : Outport  Port=7
  code_rate : Outport  Port=8
  Chan_BW : Outport  Port=9
  N_DBPS : Outport  Port=10
  N_CBPS : Outport  Port=11
  N_SS : Outport  Port=12
  HT-SIG Done : Outport  Port=13
  wires:
  rst/1 -> DOUT1/2, DOUT2/2, DOUT3/2, DOUT4/2, CRC8 Calc/4(reset), DOUT/2
  Logical1/1 -> DOUT1/3
  Logical2/1 -> DOUT/3
  Logical/1 -> DOUT2/3
  Relational/1 -> Logical1/2
  Relational2/1 -> Logical2/2
  Relational1/1 -> Logical/2
  Constant2/1 -> Relational2/2
  Constant1/1 -> Relational1/2
  Constant/1 -> Relational/2
  byte/1 -> DOUT1/1, DOUT2/1, DOUT4/1, CRC8 Calc/3(data_byte), Mux/2, DOUT3/1, DOUT/1
  byte_ind/1 -> Relational/1, Relational1/1, Relational3/1, Relational4/1, CRC8 Calc/1(byte_ind), Relational5/1, Relational2/1
  byte_valid/1 -> Logical1/1, Logical/1, Logical4/1, Logical3/1, CRC8 Calc/2(data_valid), Logical5/1, Logical2/1
  Logical4/1 -> DOUT4/3
  Logical5/1 -> DOUT3/3
  Logical3/1 -> Delay/1
  Relational3/1 -> Logical4/2, Concat2/1
  Relational5/1 -> Logical5/2
  Relational4/1 -> Logical3/2, Concat2/2
  Constant5/1 -> Relational5/2
  Constant4/1 -> Relational4/2
  Constant3/1 -> Relational3/2
  DOUT/1 -> HT-SIG Flags/1(B3), MCS Decode/1(B3)
  DOUT1/1 -> HT Length/1(B4)
  DOUT2/1 -> HT Length/2(B5)
  DOUT3/1 -> HT-SIG Flags/2(B6), MCS Decode/2(B6)
  Gateway Out1/1 -> HT-SIG Decode/1  "Length"
  Gateway Out10/1 -> HT-SIG Decode/8  "HT-SIG Valid"
  Gateway Out2/1 -> HT-SIG Decode/2  "MCS"
  Gateway Out3/1 -> HT-SIG Decode/3  "Mod Order"
  Gateway Out4/1 -> HT-SIG Decode/4  "Code Rate"
  MCS Decode/1(MCS) -> MCS/1, Gateway Out2/1
  MCS Decode/2(mod_sel) -> mod_sel/1, Gateway Out3/1
  MCS Decode/3(code_rate) -> code_rate/1, Gateway Out4/1
  MCS Decode/4(N_CBPS) -> N_CBPS/1
  MCS Decode/5(N_DBPS) -> N_DBPS/1
  MCS Decode/6(N_SS) -> N_SS/1
  MCS Decode/7(Chan_BW) -> Chan_BW/1, Gateway Out5/1
  HT Length/1(length) -> Length/1, Gateway Out1/1
  Logical6/1 -> HT-SIG Invalid/1, Gateway Out7/1
  Logical8/1 -> HT-SIG Valid/1, Gateway Out10/1
  Delay/1 -> Delay1/1
  HT-SIG Flags/1(Unsupported) -> Logical9/2
  MCS Decode/8(Unsupported) -> Gateway Out6/1, Logical9/1
  Gateway Out5/1 -> HT-SIG Decode/5  "Chan BW"
  Gateway Out6/1 -> HT-SIG Decode/6  "Unsupported"
  Delay1/1 -> HT-SIG Done/1, Logical8/2, Logical6/2
  DOUT4/1 -> HT-SIG Flags/3(B7)
  Logical9/1 -> Unsupported/1
  Gateway Out7/1 -> HT-SIG Decode/7  "HT-SIG Invalid"
  Inverter4/1 -> Logical6/1
  Mux/1 -> HT-SIG Bytes/1
  Concat2/1 -> Mux/1
  MCS Decode/9(MCS Valid) -> Inverter4/1, Logical8/1
  CRC8 Calc/1(CRC8) -> Format/1(CRC)
  Format/2(HTSIG[5]) -> Mux/3
  Format/1(HTSIG[4]) -> Mux/4

== system wlan_phy_tx_pmd/PSDU Syms Gen/Pkt Data/SIGNAL & HT-SIG Decode/S-R Latch1 ==
  S : Inport
  R : Inport  Port=2
  Constant1 : xbsIndex_r4/Constant  const=1  gui_display_data_type=Fixed-point  arith_type=Boolean  n_bits=1  bin_pt=0  preci_type=Single  exp_width=8  frac_width=24  explicit_period=off  period=1  equ=P=C  opselect=C  inp2=PCIN>>17  opr=+  inp1=P  carry=CIN  dbl_ovrd=off  block_type=constant
      settings: block_version=VER_STRING_GOES_HERE
  Convert1 : xbsIndex_r4/Convert  gui_display_data_type=Boolean  arith_type=Boolean  n_bits=1  bin_pt=0  float_type=Single  exp_bits=8  fraction_bits=24  quantization=Truncate  overflow=Wrap  en=off  latency=0  dbl_ovrd=off  pipeline=off  block_type=convert
  Convert2 : xbsIndex_r4/Convert  gui_display_data_type=Boolean  arith_type=Boolean  n_bits=1  bin_pt=0  float_type=Single  exp_bits=8  fraction_bits=24  quantization=Truncate  overflow=Wrap  en=off  latency=0  dbl_ovrd=off  pipeline=off  block_type=convert
  Register2 : xbsIndex_r4/Register  init=0  rst=on  en=on  dbl_ovrd=off  block_type=register
      settings: xl_area=[1 1 0 0 0 0 0]  block_version=VER_STRING_GOES_HERE
  Q : Outport
  wires:
  Convert2/1 -> Register2/3
  Convert1/1 -> Register2/2
  Constant1/1 -> Register2/1
  R/1 -> Convert1/1
  Register2/1 -> Q/1
  S/1 -> Convert2/1

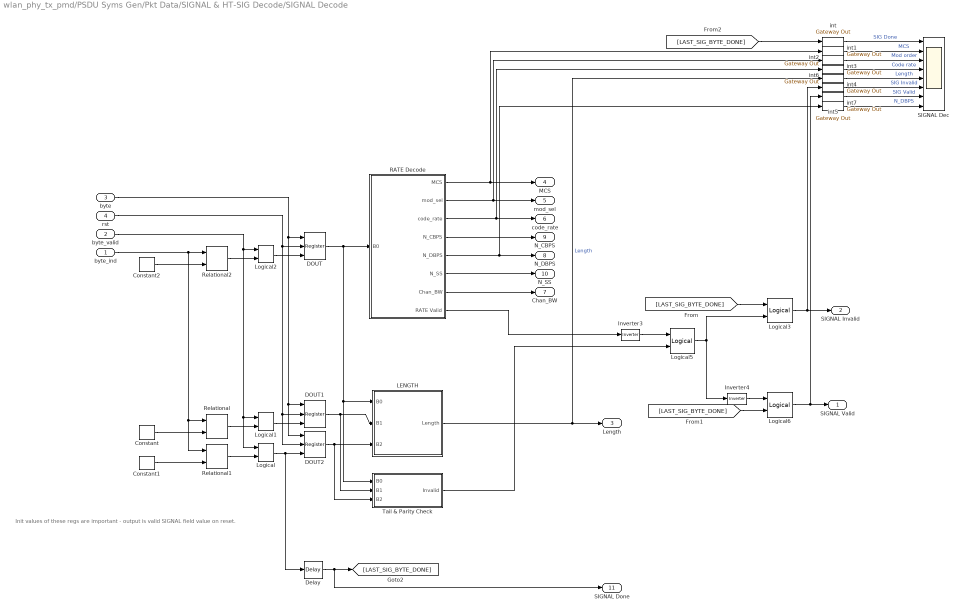
== system wlan_phy_tx_pmd/PSDU Syms Gen/Pkt Data/SIGNAL & HT-SIG Decode/SIGNAL Decode ==
  note: Init values of these regs are important - output
      | is valid SIGNAL field value on reset.
  byte_ind : Inport
  byte_valid : Inport  Port=2
  byte : Inport  Port=3
  rst : Inport  Port=4
  Constant : xbsIndex_r4/Constant  const=1  gui_display_data_type=Fixed-point  arith_type=Unsigned  n_bits=2  bin_pt=0  preci_type=Single  exp_width=8  frac_width=24  explicit_period=off  period=1  equ=P=C  opselect=C  inp2=PCIN>>17  opr=+  inp1=P  carry=CIN  dbl_ovrd=off  block_type=constant
  Constant1 : xbsIndex_r4/Constant  const=2  gui_display_data_type=Fixed-point  arith_type=Unsigned  n_bits=2  bin_pt=0  preci_type=Single  exp_width=8  frac_width=24  explicit_period=off  period=1  equ=P=C  opselect=C  inp2=PCIN>>17  opr=+  inp1=P  carry=CIN  dbl_ovrd=off  block_type=constant
  Constant2 : xbsIndex_r4/Constant  const=0  gui_display_data_type=Fixed-point  arith_type=Unsigned  n_bits=2  bin_pt=0  preci_type=Single  exp_width=8  frac_width=24  explicit_period=off  period=1  equ=P=C  opselect=C  inp2=PCIN>>17  opr=+  inp1=P  carry=CIN  dbl_ovrd=off  block_type=constant
  DOUT : xbsIndex_r4/Register  init=hex2dec('6B')  rst=on  en=on  dbl_ovrd=off  block_type=register
  DOUT1 : xbsIndex_r4/Register  init=hex2dec('07')  rst=on  en=on  dbl_ovrd=off  block_type=register
  DOUT2 : xbsIndex_r4/Register  init=hex2dec('00')  rst=on  en=on  dbl_ovrd=off  block_type=register
  Delay : xbsIndex_r4/Delay  rst=off  infoeditControl=Selection of Reset will increase slice count due to use of real FFs and instead of SRLs  en=off  latency=1  dbl_ovrd=off  reg_retiming=off  block_type=delay
  Inverter3 : xbsIndex_r4/Inverter  en=off  latency=0  dbl_ovrd=off  block_type=inv
  Inverter4 : xbsIndex_r4/Inverter  en=off  latency=0  dbl_ovrd=off  block_type=inv
  LENGTH : Subsystem
  Logical{,1..3,6} (5 alike) : xbsIndex_r4/Logical  logical_function=AND  inputs=2  en=off  latency=0  precision=Full  arith_type=Unsigned  n_bits=16  bin_pt=0  align_bp=on  dbl_ovrd=off  block_type=logical
  Logical5 : xbsIndex_r4/Logical  logical_function=OR  inputs=2  en=off  latency=0  precision=Full  arith_type=Unsigned  n_bits=16  bin_pt=0  align_bp=on  dbl_ovrd=off  block_type=logical
  RATE Decode : Subsystem
  Relational : xbsIndex_r4/Relational  mode=a=b  en=off  latency=0  dbl_ovrd=off  block_type=relational
  Relational1 : xbsIndex_r4/Relational  mode=a=b  en=off  latency=0  dbl_ovrd=off  block_type=relational
  Relational2 : xbsIndex_r4/Relational  mode=a=b  en=off  latency=0  dbl_ovrd=off  block_type=relational
  SIGNAL Dec : Scope  NumInputPorts=8
      settings: TimeRange=1000  YMin=0~-1~-1~-1~52~-1~0~0  YMax=1~1~1~1~60~1~1~30  SaveName=ScopeData18
  Tail & Parity Check : Subsystem
  int{,1..7} (8 alike) : xbsIndex_r4/Gateway Out  inherit_from_input=off  hdl_port=off  timing_constraint=None  locs_specified=off  LOCs={}  UseAsDAC=off  DACChannel='1'  block_type=gatewayout
  SIGNAL Valid : Outport
  SIGNAL Invalid : Outport  Port=2
  Length : Outport  Port=3
  MCS : Outport  Port=4
  mod_sel : Outport  Port=5
  code_rate : Outport  Port=6
  Chan_BW : Outport  Port=7
  N_DBPS : Outport  Port=8
  N_CBPS : Outport  Port=9
  N_SS : Outport  Port=10
  SIGNAL Done : Outport  Port=11
  wires:
  DOUT2/1 -> Tail & Parity Check/3(B2), LENGTH/3(B2)
  DOUT1/1 -> Tail & Parity Check/2(B1), LENGTH/2(B1)
  DOUT/1 -> Tail & Parity Check/1(B0), LENGTH/1(B0), RATE Decode/1(B0)
  rst/1 -> DOUT/2, DOUT1/2, DOUT2/2
  Logical1/1 -> DOUT1/3
  Logical2/1 -> DOUT/3
  Logical/1 -> DOUT2/3, Delay/1
  Relational/1 -> Logical1/2
  Relational2/1 -> Logical2/2
  Relational1/1 -> Logical/2
  Constant2/1 -> Relational2/2
  Constant1/1 -> Relational1/2
  Constant/1 -> Relational/2
  byte/1 -> DOUT2/1, DOUT1/1, DOUT/1
  byte_ind/1 -> Relational/1, Relational1/1, Relational2/1
  byte_valid/1 -> Logical/1, Logical1/1, Logical2/1
  Delay/1 -> [LAST_SIG_BYTE_DONE], SIGNAL Done/1
  RATE Decode/1(MCS) -> MCS/1, int1/1
  RATE Decode/2(mod_sel) -> mod_sel/1, int2/1
  RATE Decode/3(code_rate) -> code_rate/1, int3/1
  RATE Decode/4(N_CBPS) -> N_CBPS/1
  RATE Decode/5(N_DBPS) -> N_DBPS/1, int7/1
  RATE Decode/6(N_SS) -> N_SS/1
  RATE Decode/7(Chan_BW) -> Chan_BW/1
  RATE Decode/8(RATE Valid) -> Inverter3/1
  [LAST_SIG_BYTE_DONE] -> Logical3/1
  Logical3/1 -> SIGNAL Invalid/1, int4/1
  Inverter3/1 -> Logical5/1
  Tail & Parity Check/1(Invalid) -> Logical5/2
  Logical5/1 -> Logical3/2, Inverter4/1
  [LAST_SIG_BYTE_DONE] -> Logical6/2
  Inverter4/1 -> Logical6/1
  Logical6/1 -> SIGNAL Valid/1, int5/1
  LENGTH/1(Length) -> Length/1, int6/1  "Length"
  int/1 -> SIGNAL Dec/1  "SIG Done"
  [LAST_SIG_BYTE_DONE] -> int/1
  int2/1 -> SIGNAL Dec/3  "Mod order"
  int1/1 -> SIGNAL Dec/2  "MCS"
  int3/1 -> SIGNAL Dec/4  "Code rate"
  int4/1 -> SIGNAL Dec/6  "SIG Invalid"
  int5/1 -> SIGNAL Dec/7  "SIG Valid"
  int6/1 -> SIGNAL Dec/5  "Length"
  int7/1 -> SIGNAL Dec/8  "N_DBPS"

== system wlan_phy_tx_pmd/PSDU Syms Gen/Pkt Data/Scrambling/Scrambling LFSR ==
  note: The standard suggests setting the state of the Tx LFSR to a pseudo-random value for
      | each new transmission. We implement this by not resetting the LFSR state between
      | transmissions. The reset-per-packet can be enabled by software if required by
      | a custom application (i.e. if you need to generate the same waveform for a given
      | payload many times).
  en : Inport
  Assert : xbsIndex_r4/Assert  assert_type=on  type_source=Explicitly  gui_display_data_type=Boolean  arith_type=Boolean  n_bits=16  bin_pt=14  preci_type=Single  exp_width=8  frac_width=24  assert_rate=on  rate_source=Explicitly  period=1  output_port=on  block_type=assert
      settings: block_version=VER_STRING_GOES_HERE
  Assert1 : xbsIndex_r4/Assert  assert_type=on  type_source=Explicitly  gui_display_data_type=Fixed-point  arith_type=Boolean  n_bits=16  bin_pt=14  preci_type=Single  exp_width=8  frac_width=24  assert_rate=on  rate_source=Explicitly  period=1  output_port=on  block_type=assert
      settings: infoedit=Asserts a user-defined sample rate and/or type on a signal.<P><P>Hardware notes: In hardware this block costs nothing.  block_version=VER_STRING_GOES_HERE
  Convert : xbsIndex_r4/Convert  gui_display_data_type=Boolean  arith_type=Boolean  n_bits=16  bin_pt=14  float_type=Single  exp_bits=8  fraction_bits=24  quantization=Truncate  overflow=Wrap  en=off  latency=0  dbl_ovrd=off  pipeline=off  block_type=convert
  Convert1 : xbsIndex_r4/Convert  gui_display_data_type=Boolean  arith_type=Boolean  n_bits=16  bin_pt=14  float_type=Single  exp_bits=8  fraction_bits=24  quantization=Truncate  overflow=Wrap  en=off  latency=0  dbl_ovrd=off  pipeline=off  block_type=convert
  Convert2 : xbsIndex_r4/Convert  gui_display_data_type=Fixed-point  arith_type=Unsigned  n_bits=1  bin_pt=0  float_type=Single  exp_bits=8  fraction_bits=24  quantization=Truncate  overflow=Wrap  en=off  latency=0  dbl_ovrd=off  pipeline=off  block_type=convert
  Logical : xbsIndex_r4/Logical  logical_function=XOR  inputs=2  en=off  latency=0  precision=Full  arith_type=Unsigned  n_bits=8  bin_pt=2  align_bp=on  dbl_ovrd=off  block_type=logical
      settings: xl_area=[0, 0, 0, 0, 0, 0, 0]  block_version=VER_STRING_GOES_HERE
  Logical1 : xbsIndex_r4/Logical  logical_function=AND  inputs=2  en=off  latency=0  precision=Full  arith_type=Unsigned  n_bits=8  bin_pt=2  align_bp=on  dbl_ovrd=off  block_type=logical
      settings: xl_area=[0, 0, 0, 0, 0, 0, 0]  block_version=VER_STRING_GOES_HERE
  Register{,1..6} (7 alike) : xbsIndex_r4/Register  init=1  rst=on  en=on  dbl_ovrd=off  block_type=register
      settings: xl_area=[0, 0, 0, 0, 0, 0, 0]  block_version=VER_STRING_GOES_HERE
  Q : Outport
  wires:
  Logical1/1 -> Convert/1
  Register6/1 -> Assert/1
  Logical/1 -> Convert2/1, Register/1
  Register5/1 -> Register6/1
  Register4/1 -> Register5/1
  Register3/1 -> Assert1/1, Register4/1
  Register2/1 -> Register3/1
  Register1/1 -> Register2/1
  Register/1 -> Register1/1
  Assert/1 -> Logical/1
  Assert1/1 -> Logical/2
  en/1 -> Convert1/1
  Convert/1 -> Register5/2, Register6/2, Register4/2, Register3/2, Register2/2, Register1/2, Register/2
  Convert1/1 -> Register5/3, Register6/3, Register4/3, Register3/3, Register2/3, Register1/3, Register/3
  Convert2/1 -> Q/1
  [TX_RESET] -> Logical1/1
  [regTx_Reset_Scrambling_LFSR_PerPkt] -> Logical1/2

== system wlan_phy_tx_pmd/PSDU Syms Gen/Puncture & Interleave/Interleaver Ctrl & Puncturing/Bit Index Calc ==
  note: Accumulator increments by 1 or 2 bits per cycle, depending
      | on whether current bit pair has a punctured value.
      | Outputs are used as memory addresses for the interleaver RAM.
  Inc : Inport
  Rst : Inport  Port=2
  En : Inport  Port=3
  Accumulator : xbsIndex_r4/Accumulator  operation=Add  n_bits=ceil(log2(MAX_NCBPS))  overflow=Wrap  scale=1  rst=on  infoeditControl=reset for floating point data type must be asserted for a minimum of 2 cycles  hasbypass=off  en=on  latency=0  dbl_ovrd=off  msb_inp=100  msb=100  lsb=-100  use_behavioral_HDL=on  implementation=Fabric  block_type=accum
  AddSub : xbsIndex_r4/AddSub  mode=Addition  use_carryin=off  use_carryout=off  en=off  latency=0  precision=User Defined  arith_type=Unsigned  n_bits=ceil(log2(MAX_NCBPS))  bin_pt=0  quantization=Truncate  overflow=Wrap  dbl_ovrd=off  use_behavioral_HDL=off  hw_selection=Fabric  pipelined=off  block_type=addsub
  Constant2 : xbsIndex_r4/Constant  const=1  gui_display_data_type=Fixed-point  arith_type=Unsigned  n_bits=1  bin_pt=0  preci_type=Single  exp_width=8  frac_width=24  explicit_period=off  period=1  equ=P=C  opselect=C  inp2=PCIN>>17  opr=+  inp1=P  carry=CIN  dbl_ovrd=off  block_type=constant
  Ind A : Outport
  Ind B : Outport  Port=2
  wires:
  Accumulator/1 -> AddSub/1, Ind A/1
  AddSub/1 -> Ind B/1
  Constant2/1 -> AddSub/2
  Rst/1 -> Accumulator/2
  En/1 -> Accumulator/3
  Inc/1 -> Accumulator/1
